simulink model "evin_model"  (R2025a)
settings: Solver=VariableStepAuto  StartTime=0.0  StopTime=inf  RelTol=1e-3
values from neighbouring files (symbols this model uses):
  A = 2    [evin_parameters.m]    (also in parameters.m)
  c_1 = 0.86    [evin_parameters.m]    (also in parameters.m)
  c_2 = 33.82    [evin_parameters.m]    (also in parameters.m)
  c_3 = 0.36    [evin_parameters.m]    (also in parameters.m)
  c_w = 0.3    [evin_parameters.m]
  g = 9.81    [evin_parameters.m]    (also in parameters.m)
  J_R = 0.8    [evin_parameters.m]
  m = 1500    [evin_parameters.m]    (also in parameters.m)
  r_R = 0.3    [evin_parameters.m]
  rho = 1.2    [evin_parameters.m]    (also in parameters.m)
  v_F0 = 100    [evin_parameters.m]
  x_F0 = 0    [evin_parameters.m]
libraries: simulink x1
settings Model: Creator=evinb  LastModifiedBy=kavin

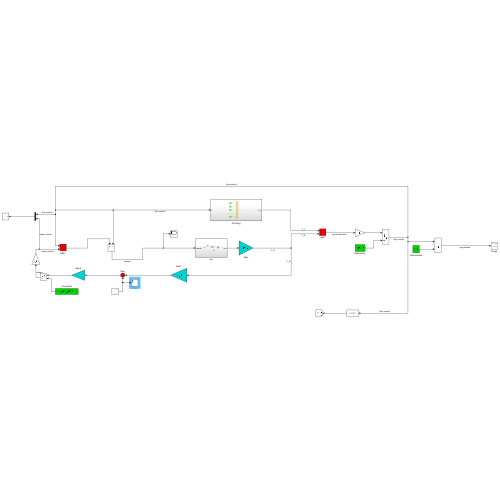
[thumbnail: Simulink's stored preview of the top-level diagram]
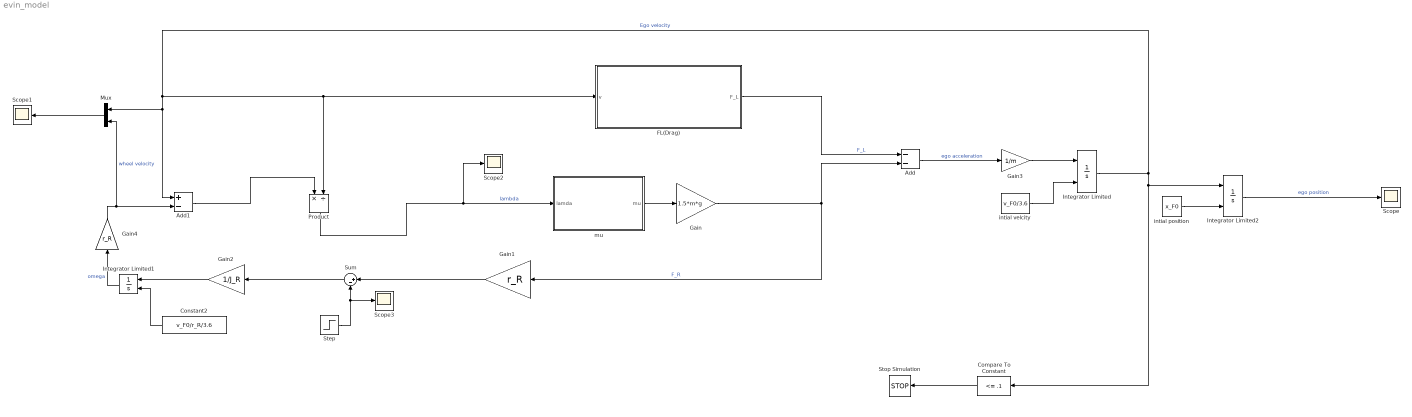
== system evin_model ==
  Add : Sum  Inputs=--
  Add1 : Sum  Inputs=+-
  Compare To Constant : simulink/Logic and Bit Operations/Compare To Constant  relop=<=  const=.1  OutDataTypeStr=boolean
  Constant2 : Constant  Value=v_F0/r_R/3.6
  FL(Drag) : Subsystem
  Gain : Gain  Gain=1.5*m*g
  Gain1 : Gain  Gain=r_R
  Gain2 : Gain  Gain=1/J_R
  Gain3 : Gain  Gain=1/m
  Gain4 : Gain  Gain=r_R
  Integrator Limited : Integrator  InitialConditionSource=external  LimitOutput=on  LowerSaturationLimit=0
  Integrator Limited1 : Integrator  InitialConditionSource=external  LimitOutput=on  LowerSaturationLimit=0
  Integrator Limited2 : Integrator  InitialConditionSource=external  LimitOutput=on  LowerSaturationLimit=0
  Mux : Mux  Inputs=2
  Product : Product  Inputs=*/
  Scope{,1..3} (4 alike) : Scope
      Scope settings: ActiveDisplayYMinimum=-0.53013516244378511  ActiveDisplayYMaximum=3.297709992621856
      Scope1 settings: ActiveDisplayYMinimum=-1.8169313409954952  ActiveDisplayYMaximum=122.57162402273404
      Scope2 settings: ActiveDisplayYMinimum=-171.20863808787055  ActiveDisplayYMaximum=19.023182009763392  DataLoggingVariableName=ScopeData2
      Scope3 settings: ActiveDisplayYMinimum=-1  ActiveDisplayYMaximum=1  DataLoggingVariableName=ScopeData3
  Step : Step  After=5355  SampleTime=0
  Stop Simulation : Stop
  Sum : Sum  Inputs=|+-
  intial position : Constant  Value=x_F0
  "intial velcity " : Constant  Value=v_F0/3.6
  mu : Subsystem
  wires:
  FL(Drag)/1(F_L) -> Add/1  "F_L"
  "intial velcity "/1 -> Integrator Limited/2
  Add/1 -> Gain3/1  "ego acceleration"
  Integrator Limited/1 -> Compare To Constant/1, Integrator Limited2/1, Mux/1, Add1/1, Product/2, FL(Drag)/1(v)  "Ego velocity"
  intial position/1 -> Integrator Limited2/2
  Integrator Limited2/1 -> Scope/1  "ego position"
  Gain/1 -> Gain1/1, Add/2  "F_R"
  mu/1(mu) -> Gain/1
  Gain1/1 -> Sum/1
  Step/1 -> Scope3/1, Sum/2
  Sum/1 -> Gain2/1
  Gain2/1 -> Integrator Limited1/1
  Constant2/1 -> Integrator Limited1/2
  Integrator Limited1/1 -> Gain4/1  "omega"
  Add1/1 -> Product/1
  Product/1 -> Scope2/1, mu/1(lamda)  "lambda"
  Gain3/1 -> Integrator Limited/1
  Compare To Constant/1 -> Stop Simulation/1
  Mux/1 -> Scope1/1
  Gain4/1 -> Mux/2, Add1/2  "wheel velocity"

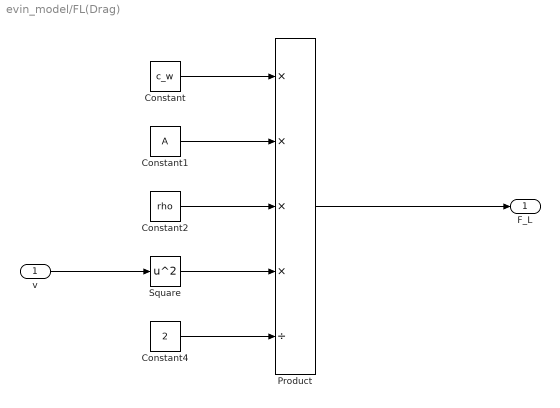
== system evin_model/FL(Drag) ==
  v : Inport
  Constant : Constant  Value=c_w
  Constant1 : Constant  Value=A
  Constant2 : Constant  Value=rho
  Constant4 : Constant  Value=2
  Product : Product  Inputs=****/
  Square : Math  Operator=square
  F_L : Outport
  wires:
  Product/1 -> F_L/1
  Square/1 -> Product/4
  Constant/1 -> Product/1
  Constant4/1 -> Product/5
  Constant2/1 -> Product/3
  Constant1/1 -> Product/2
  v/1 -> Square/1

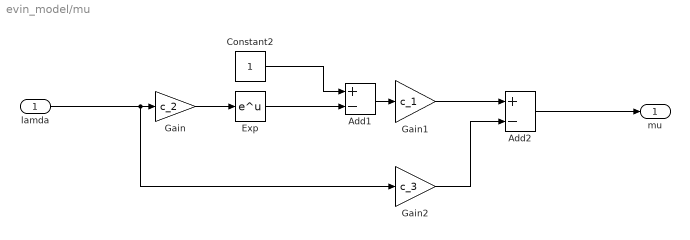
== system evin_model/mu ==
  lamda : Inport
  Add1 : Sum  Inputs=+-
  Add2 : Sum  Inputs=+-
  Constant2 : Constant
  Exp : Math
  Gain : Gain  Gain=c_2
  Gain1 : Gain  Gain=c_1
  Gain2 : Gain  Gain=c_3
  mu : Outport
  wires:
  Add2/1 -> mu/1
  Exp/1 -> Add1/2
  Gain2/1 -> Add2/2
  Gain1/1 -> Add2/1
  Add1/1 -> Gain1/1
  Constant2/1 -> Add1/1
  lamda/1 -> Gain2/1, Gain/1
  Gain/1 -> Exp/1
